simulink model "MSD_sim_sol"  (R2023b)
settings: Solver=ode3  StartTime=0.0  StopTime=15  FixedStep=0.01  RelTol=1e-3
values from neighbouring files (symbols this model uses):
  a_vect = [ k ; d ; m ]    [MSD_par_sol.m]    (also in balloon_par_sol.m = -At(3,:)'; dmass_par_sol.m = -At(4,1:4)')
  alpha_vect = poly3traj([p0;v0],[pT;vT],H)    [MSD_par_sol.m]    (also in balloon_par_sol.m = poly5traj([h0;v0;a0],[hT;vT;aT],T); dmass_par_sol.m = poly7traj(z0,zT,H))
  d = 0.1    [MSD_par_sol.m]
  k = 5    [MSD_par_sol.m]    (also in dmass_par_sol.m)
  m = 10    [MSD_par_sol.m]
  ustar = k*pT    (= 150)    [MSD_par_sol.m]
settings Model: Creator=jerome  LastModifiedBy=jerome
settings ModelReferenceCC: EnableRefExpFcnMdlSchedulingChecks=on

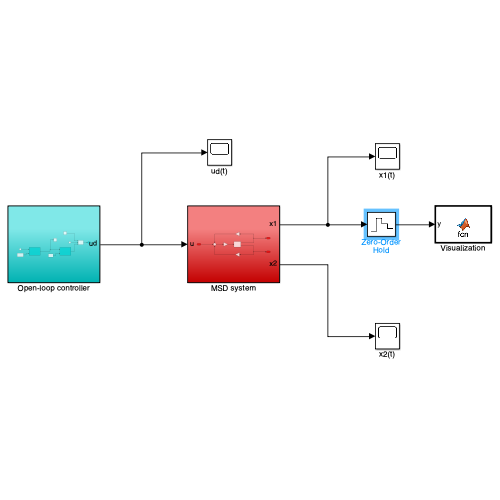
[thumbnail: Simulink's stored preview of the top-level diagram]
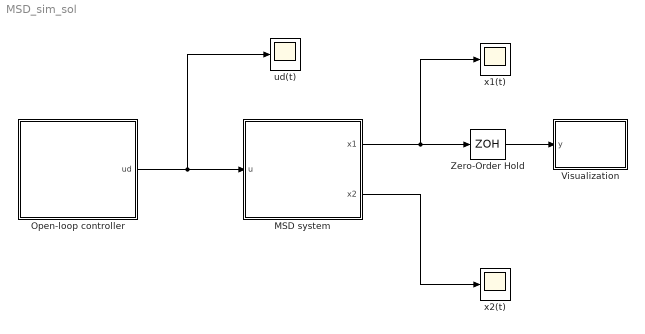
== system MSD_sim_sol ==
  MSD system : Subsystem
  Open-loop controller : Subsystem
  Visualization : MATLAB Function  TreatAsAtomicUnit=on
  Zero-Order Hold : ZeroOrderHold  SampleTime=0.2
  ud(t) : Scope
  x1(t) : Scope
  x2(t) : Scope
  wires:
  Open-loop controller/1(ud) -> ud(t)/1, MSD system/1(u)
  MSD system/2(x2) -> x2(t)/1
  MSD system/1(x1) -> x1(t)/1, Zero-Order Hold/1
  Zero-Order Hold/1 -> Visualization/1(y)

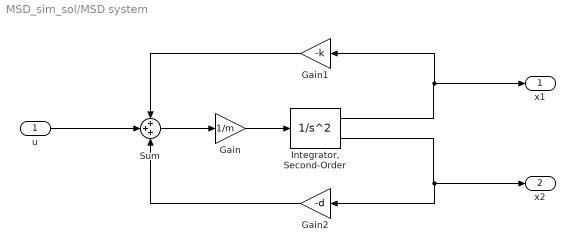
== system MSD_sim_sol/MSD system ==
  u : Inport
  Gain : Gain  Gain=1/m
  Gain1 : Gain  Gain=-k
  Gain2 : Gain  Gain=-d
  "Integrator, Second-Order" : SecondOrderIntegrator
  Sum : Sum  Inputs=+++
  x1 : Outport
  x2 : Outport  Port=2
  wires:
  "Integrator, Second-Order"/1 -> Gain1/1, x1/1
  "Integrator, Second-Order"/2 -> Gain2/1, x2/1
  Gain/1 -> "Integrator, Second-Order"/1
  Sum/1 -> Gain/1
  u/1 -> Sum/2
  Gain1/1 -> Sum/1
  Gain2/1 -> Sum/3

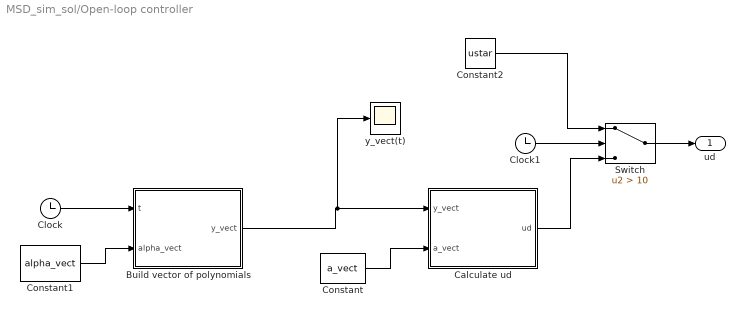
== system MSD_sim_sol/Open-loop controller ==
  Build vector of polynomials : MATLAB Function  TreatAsAtomicUnit=on
  Calculate ud : MATLAB Function  TreatAsAtomicUnit=on
  Clock : Clock
  Clock1 : Clock
  Constant : Constant  Value=a_vect  VectorParams1D=off
  Constant1 : Constant  Value=alpha_vect  VectorParams1D=off
  Constant2 : Constant  Value=ustar
  Switch : Switch  Criteria=u2 > Threshold  Threshold=10  SaturateOnIntegerOverflow=off  InputSameDT=off
  y_vect(t) : Scope
  ud : Outport
  wires:
  Build vector of polynomials/1(y_vect) -> y_vect(t)/1, Calculate ud/1(y_vect)
  Constant/1 -> Calculate ud/2(a_vect)
  Constant1/1 -> Build vector of polynomials/2(alpha_vect)
  Clock/1 -> Build vector of polynomials/1(t)
  Calculate ud/1(ud) -> Switch/3
  Switch/1 -> ud/1
  Clock1/1 -> Switch/2
  Constant2/1 -> Switch/1

== matlab function MSD_sim_sol/Open-loop controller/Calculate ud ==
  data: y_vect input; ud output; a_vect input
function ud = fcn(y_vect,a_vect)

ae_vect = [ a_vect ; 1 ];


% computation open-loop input
ud = a_vect' * y_vect;

== matlab function MSD_sim_sol/Visualization ==
  data: y input
function fcn(y)


% the mass
    Xmass = [ 5 ; 5 ; -5 ; -5 ; 5 ] + y;
    Ymass = [ -5 ; 5 ; 5 ; -5 ; -5]; 

% the spring
    Xspring = [ 0 ; 4 ; 6 ; 10 ; 14 ; 18 ; 20 ; 24 ]/24*(y+24) - 29;
    Yspring = [ 0 ; 0 ; 3 ; -3 ; 3 ; -3 ; 0 ; 0 ];

% to be able to use 'fill' even though the function is not supported for code generation
% see https://se.mathworks.com/help/simulink/slref/coder.extrinsic.html
coder.extrinsic('fill'); 

% draw the mass of the MSD system
fill(Xmass,Ymass,'r');

hold on
% draw the spring
plot(Xspring,Yspring,'b','Linewidth',3);

% draw misc
plot([-29 -29],[-10 10],'k','Linewidth',3); %draw a thick line on the left
plot([0 0],[-10 -7],'k','Linewidth',2);  %draw a thin line at position x = 0

hold off

axis([-40 40 -10 10]);
title('Mass-Spring-Damper system', 'FontSize',20);
axis equal;
grid on;

drawnow;

== matlab function MSD_sim_sol/Open-loop controller/Build vector of polynomials ==
  data: t input; y_vect output; alpha_vect input
function y_vect = fcn(t,alpha_vect)

if length(alpha_vect) == 4
    t_vect0 = [ 1 ; t ; t^2 ; t^3 ]; % vector of t values
    t_vect1 = [ 0 ; 1 ; 2*t ; 3*t^2 ]; % derivative of t_vect0
    t_vect2 = [ 0 ; 0 ; 2 ; 2*3*t ]; % derivative of t_vect1
elseif length(alpha_vect) == 6
    t_vect0 = [ 1 ; t ; t^2 ; t^3 ; t^4 ; t^5 ]; % vector of t values
    t_vect1 = [ 0 ; 1 ; 2*t ; 3*t^2 ; 4*t^3 ; 5*t^4 ]; % derivative of t_vect0
    t_vect2 = [ 0 ; 0 ; 2 ; 2*3*t ; 3*4*t^2 ; 4*5*t^3 ]; % derivative of t_vect1
else 
    t_vect0 = [ 1 ; t ; t^2 ; t^3 ; t^4 ; t^5 ; t^6 ; t^7 ]; % vector of t values
    t_vect1 = [ 0 ; 1 ; 2*t ; 3*t^2 ; 4*t^3 ; 5*t^4 ; 6*t^5 ; 7*t^6 ]; % derivative of t_vect0
    t_vect2 = [ 0 ; 0 ; 2 ; 2*3*t ; 3*4*t^2 ; 4*5*t^3 ; 5*6*t^4 ; 6*7*t^5 ]; % derivative of t_vect1
end


yd = t_vect0'*alpha_vect;
yd_dot = t_vect1'*alpha_vect;
yd_ddot = t_vect2'*alpha_vect;

% vector of desired trajectory and its derivatives
y_vect = [ yd ; yd_dot ; yd_ddot ];
